simulink model "axes_delay"  (R2021b)
settings: Solver=FixedStepDiscrete  StartTime=0.0  StopTime=inf  FixedStep=0.1  RelTol=1e-3
undefined symbols (not defined in the file): Levenberg, Marquardt, W, X, Y, Z
libraries: robotlib x7, simulink x2, robotmaniplib x2, robotcorelib x1
settings Model: Creator=alessandrini  LastModifiedBy=alessandrini
settings OptimizationCC: EnhancedBackFolding=on  PassReuseOutputArgsAs=Individual arguments  ZeroExternalMemoryAtStartup=off  ZeroInternalMemoryAtStartup=off  MaxStackSize=64  OptimizeBlockOrder=speed  DifferentSizesBufferReuse=on  OptimizationCustomize=off  EfficientTunableParamExpr=on
settings DebuggingCC: ParameterTunabilityLossMsg=error
settings HardwareCC: ProdBitPerPointer=32  ProdBitPerSizeT=32  ProdBitPerPtrDiffT=32  ProdLargestAtomicFloat=None  ProdIntDivRoundTo=Undefined  ProdEndianess=Unspecified  ProdWordSize=32  ProdHWDeviceType=Generic->Unspecified (assume 32-bit Generic)  UseEmbeddedCoderFeatures=off
settings RTWCC: Description=Embedded Coder  SystemTargetFile=ert.tlc  HardwareBoard=Robot Operating System (ROS)  TLCOptions="-aInlineSetEventsForThisBaseRateFcn=TLC_FALSE -aSuppressMultiTaskScheduler=TLC_FALSE  -aRateBasedStepFcn=0"  TemplateMakefile=ert_default_tmf  Toolchain=Catkin  TargetLang=C++
settings CodeAppCC: ForceParamTrailComments=on  IgnoreCustomStorageClasses=off  OperatorAnnotations=on  SimulinkDataObjDesc=on  SFDataObjDesc=on  InsertBlockDesc=on
settings ERTTargetCC: SupportNonInlinedSFcns=on

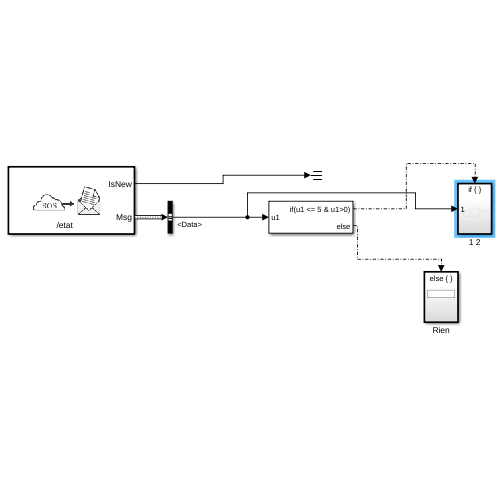
[thumbnail: Simulink's stored preview of the top-level diagram]
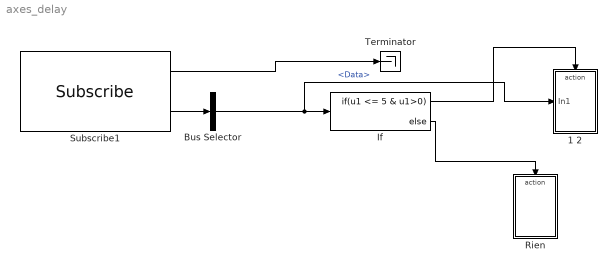
== system axes_delay ==
  1 2 : Subsystem
  Bus Selector : BusSelector  OutputSignals=Data
  If : If  IfExpression=u1 <= 5 & u1>0
  Rien : Subsystem
  Subscribe1 : robotlib/Subscribe  topicSource=Specify your own  topic=/etat  messageType=std_msgs/Int16  SampleTime=-1  legacyBusStruct=off  messageQueueLength=1
  Terminator : Terminator
  wires:
  If/1 -> 1 2/Action
  If/2 -> Rien/Action
  Subscribe1/1 -> Terminator/1
  Subscribe1/2 -> Bus Selector/1
  Bus Selector/1 -> 1 2/1(In1), If/1  "<Data>"

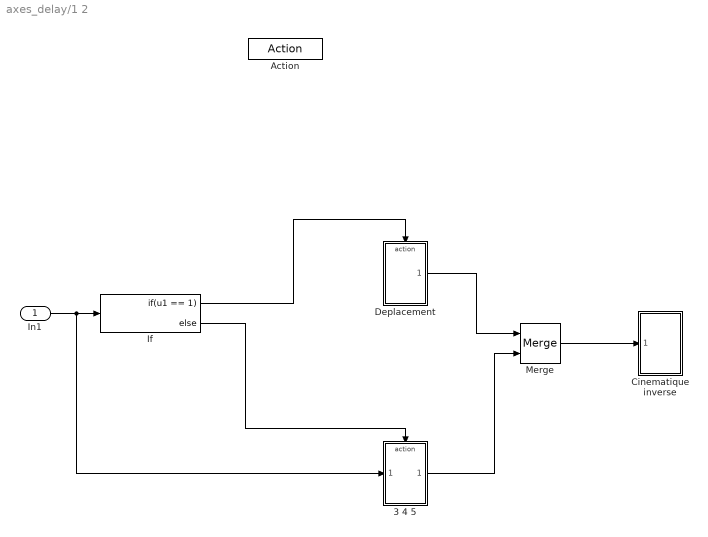
== system axes_delay/1 2 ==
  In1 : Inport
  Action : ActionPort  InitializeStates=reset  ActionPortLabel=if(u1 <= 5 & u1>0)
  3 4 5 : Subsystem
  Cinematique inverse : Subsystem
  Deplacement : Subsystem
  If : If  IfExpression=u1 == 1
  Merge : Merge
  wires:
  Merge/1 -> Cinematique inverse/1(position_robot)
  In1/1 -> 3 4 5/1(In1), If/1
  If/1 -> Deplacement/Action
  If/2 -> 3 4 5/Action
  3 4 5/1(position_robot) -> Merge/2
  Deplacement/1(position_robot) -> Merge/1

== system axes_delay/Rien ==
  Action : ActionPort  InitializeStates=reset  ActionPortLabel=else

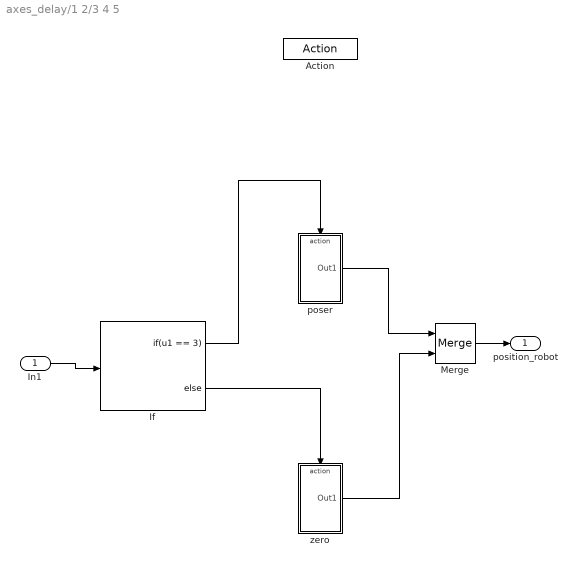
== system axes_delay/1 2/3 4 5 ==
  In1 : Inport
  Action : ActionPort  InitializeStates=reset  ActionPortLabel=else
  If : If  IfExpression=u1 == 3
  Merge : Merge
  poser : Subsystem
  zero : Subsystem
  position_robot : Outport
  wires:
  If/2 -> zero/Action
  In1/1 -> If/1
  If/1 -> poser/Action
  zero/1(Out1) -> Merge/2
  poser/1(Out1) -> Merge/1
  Merge/1 -> position_robot/1

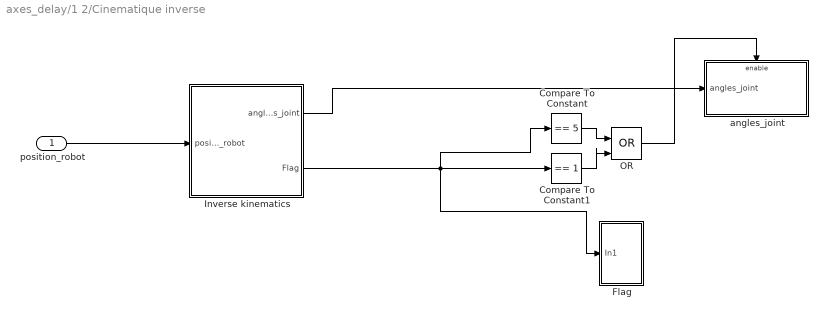
== system axes_delay/1 2/Cinematique inverse ==
  position_robot : Inport
  Compare To Constant : simulink/Logic and Bit Operations/Compare To Constant  relop===  const=5  OutDataTypeStr=boolean
  Compare To Constant1 : simulink/Logic and Bit Operations/Compare To Constant  relop===  const=1  OutDataTypeStr=boolean
  Flag : Subsystem
  Inverse kinematics : Subsystem
  OR : Logic  Operator=OR  IconShape=distinctive  AllPortsSameDT=off  OutDataTypeStr=boolean
  angles_joint : Subsystem
  wires:
  OR/1 -> angles_joint/Enable
  Compare To Constant/1 -> OR/1
  Compare To Constant1/1 -> OR/2
  Inverse kinematics/2(Flag) -> Flag/1(In1), Compare To Constant/1, Compare To Constant1/1
  position_robot/1 -> Inverse kinematics/1(position_robot)
  Inverse kinematics/1(angles_joint) -> angles_joint/1(angles_joint)

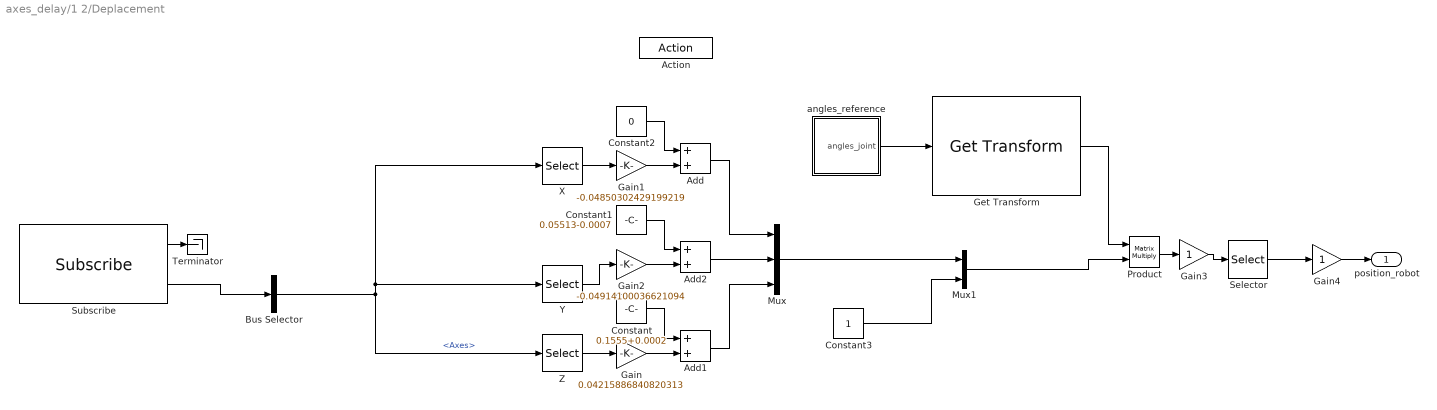
== system axes_delay/1 2/Deplacement ==
  Action : ActionPort  InitializeStates=reset  ActionPortLabel=if(u1 == 1)
  Add : Sum
  Add1 : Sum
  Add2 : Sum
  Bus Selector : BusSelector  OutputSignals=Axes
  Constant : Constant  Value=0.1555+0.0002
  Constant1 : Constant  Value=0.05513-0.0007
  Constant2 : Constant  Value=0
  Constant3 : Constant
  Gain : Gain  Gain=0.04215886840820313
  Gain1 : Gain  Gain=-0.04850302429199219
  Gain2 : Gain  Gain=-0.04914100036621094
  Gain3 : Gain
  Gain4 : Gain
  Get Transform : robotmaniplib/Get Transform  RigidBodyTree=robot  SourceBody=Body6  TargetBody=Base  SimulateUsing=Interpreted execution
  Mux : Mux  Inputs=3
  Mux1 : Mux  Inputs=2
  Product : Product  Multiplication=Matrix(*)
  Selector : Selector  InputPortWidth=4  IndexOptions=Starting index (dialog)  Indices=[1]  OutputSizes=3
  Subscribe : robotlib/Subscribe  topicSource=Select from ROS network  topic=/joy  messageType=sensor_msgs/Joy  SampleTime=-1  legacyBusStruct=off  messageQueueLength=1
  Terminator : Terminator
  X : Selector  InputPortWidth=128  IndexOptions=Index vector (dialog)  Indices=[4]  OutputSizes=1
  Y : Selector  InputPortWidth=128  IndexOptions=Index vector (dialog)  Indices=[5]  OutputSizes=1
  Z : Selector  InputPortWidth=128  IndexOptions=Index vector (dialog)  Indices=[2]  OutputSizes=1
  angles_reference : Subsystem
  position_robot : Outport
  wires:
  Gain2/1 -> Add2/2
  Mux/1 -> Mux1/1
  X/1 -> Gain1/1
  Selector/1 -> Gain4/1
  Constant/1 -> Add1/1
  Bus Selector/1 -> X/1, Y/1, Z/1  "<Axes>"
  Mux1/1 -> Product/2
  Add/1 -> Mux/1
  Subscribe/2 -> Bus Selector/1
  Gain/1 -> Add1/2
  Get Transform/1 -> Product/1
  Constant1/1 -> Add2/1
  angles_reference/1(angles_joint) -> Get Transform/1
  Gain1/1 -> Add/2
  Gain4/1 -> position_robot/1
  Gain3/1 -> Selector/1
  Add1/1 -> Mux/3
  Constant3/1 -> Mux1/2
  Product/1 -> Gain3/1
  Z/1 -> Gain/1
  Y/1 -> Gain2/1
  Constant2/1 -> Add/1
  Add2/1 -> Mux/2
  Subscribe/1 -> Terminator/1

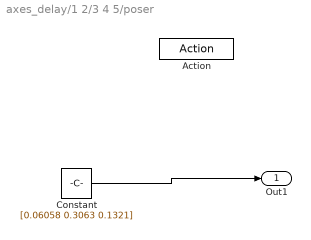
== system axes_delay/1 2/3 4 5/poser ==
  Action : ActionPort  InitializeStates=reset  ActionPortLabel=if(u1 == 3)
  Constant : Constant  Value=[0.06058 0.3063 0.1321]
  Out1 : Outport
  wires:
  Constant/1 -> Out1/1

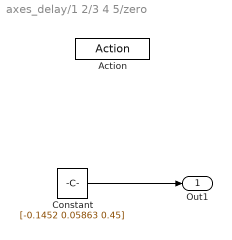
== system axes_delay/1 2/3 4 5/zero ==
  Action : ActionPort  InitializeStates=reset  ActionPortLabel=else
  Constant : Constant  Value=[-0.1452 0.05863 0.45]
  Out1 : Outport
  wires:
  Constant/1 -> Out1/1

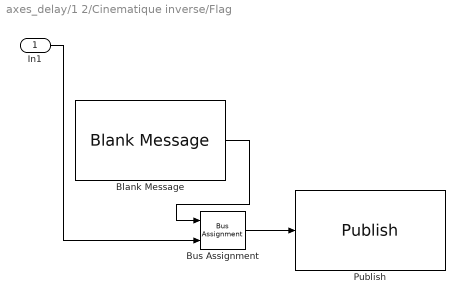
== system axes_delay/1 2/Cinematique inverse/Flag ==
  In1 : Inport
  Blank Message : robotlib/Blank Message  messageClass=Message  entityType=std_msgs/UInt16  messageType=std_msgs/UInt16  SampleTime=-1  legacyBusStruct=off
  Bus Assignment : BusAssignment  AssignedSignals=Data
  Publish : robotlib/Publish  topicSource=Specify your own  topic=/flag  messageType=std_msgs/UInt16  legacyBusStruct=off  messageQueueLength=1
  wires:
  Bus Assignment/1 -> Publish/1
  In1/1 -> Bus Assignment/2
  Blank Message/1 -> Bus Assignment/1

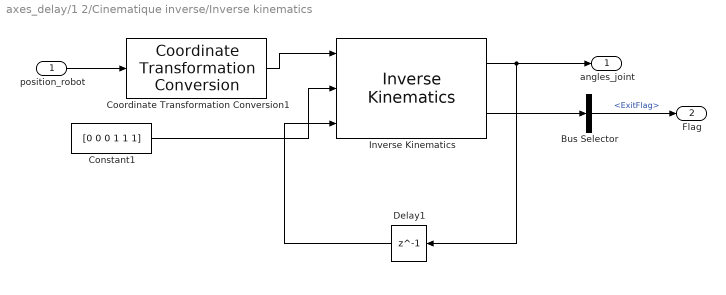
== system axes_delay/1 2/Cinematique inverse/Inverse kinematics ==
  position_robot : Inport
  Bus Selector : BusSelector  OutputSignals=ExitFlag
  Constant1 : Constant  Value=[0 0 0 1 1 1]  VectorParams1D=off
  Coordinate Transformation Conversion1 : robotcorelib/Coordinate Transformation Conversion  InputRepresentation=Translation Vector  InputEulerSequence=ZYX  ShowTrVecInputPort=on  OutputRepresentation=Homogeneous Transformation  OutputEulerSequence=ZYX  ShowTrVecOutputPort=on  SimulateUsing=Interpreted execution
  Delay1 : Delay  DelayLength=1  InitialCondition=([19 43 0 -30]*pi/180)'  SampleTime=0.1
  Inverse Kinematics : robotmaniplib/Inverse Kinematics  RigidBodyTree=robot  EndEffector=Body5  ShowInfo=on  SolverName=Levenberg-Marquardt  EnforceJointLimits=on  MaxIterations=1500  MaxTime=10  GradientTolerance=1e-7  SolutionTolerance=1e-6  StepTolerance=1e-14  ErrorChangeTolerance=1e-12  UseErrorDamping=on  DampingBias=0.0025  SimulateUsing=Interpreted execution
  angles_joint : Outport
  Flag : Outport  Port=2
  wires:
  Inverse Kinematics/1 -> Delay1/1, angles_joint/1
  Inverse Kinematics/2 -> Bus Selector/1
  position_robot/1 -> Coordinate Transformation Conversion1/1
  Constant1/1 -> Inverse Kinematics/2
  Coordinate Transformation Conversion1/1 -> Inverse Kinematics/1
  Delay1/1 -> Inverse Kinematics/3
  Bus Selector/1 -> Flag/1  "<ExitFlag>"

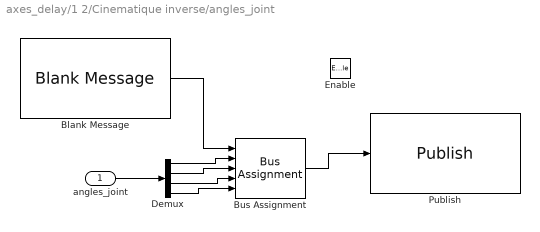
== system axes_delay/1 2/Cinematique inverse/angles_joint ==
  angles_joint : Inport
  Enable : EnablePort
  Blank Message : robotlib/Blank Message  messageClass=Message  entityType=geometry_msgs/Quaternion  messageType=geometry_msgs/Quaternion  SampleTime=-1  legacyBusStruct=off
  Bus Assignment : BusAssignment  AssignedSignals=X,Y,Z,W
  Demux : Demux
  Publish : robotlib/Publish  topicSource=Specify your own  topic=/angles_joint_limit  messageType=geometry_msgs/Quaternion  legacyBusStruct=off  messageQueueLength=1
  wires:
  Bus Assignment/1 -> Publish/1
  Blank Message/1 -> Bus Assignment/1
  Demux/4 -> Bus Assignment/5
  Demux/3 -> Bus Assignment/4
  Demux/2 -> Bus Assignment/3
  Demux/1 -> Bus Assignment/2
  angles_joint/1 -> Demux/1

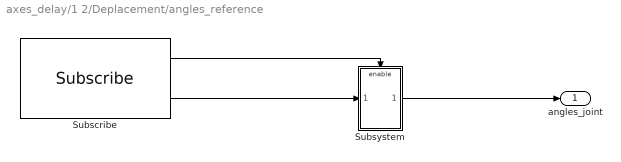
== system axes_delay/1 2/Deplacement/angles_reference ==
  Subscribe : robotlib/Subscribe  topicSource=Specify your own  topic=/angles_joint  messageType=geometry_msgs/Quaternion  SampleTime=-1  legacyBusStruct=off  messageQueueLength=1
  Subsystem : Subsystem
  angles_joint : Outport
  wires:
  Subscribe/2 -> Subsystem/1(In1)
  Subsystem/1(Out1) -> angles_joint/1
  Subscribe/1 -> Subsystem/Enable

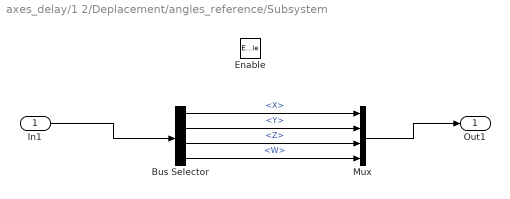
== system axes_delay/1 2/Deplacement/angles_reference/Subsystem ==
  In1 : Inport
  Enable : EnablePort
  Bus Selector : BusSelector  OutputSignals=X,Y,Z,W
  Mux : Mux
  Out1 : Outport
  wires:
  In1/1 -> Bus Selector/1
  Bus Selector/2 -> Mux/2  "<Y>"
  Bus Selector/1 -> Mux/1  "<X>"
  Mux/1 -> Out1/1
  Bus Selector/3 -> Mux/3  "<Z>"
  Bus Selector/4 -> Mux/4  "<W>"
